simulink model "sddac"  (Simulink 5.0)
settings: Solver=ode45  StartTime=0.0  StopTime=10.0  RelTol=1e-3
values from neighbouring files (symbols this model uses):
  C = 680e-9    (= 6.8e-07)    [DPLL_init_2.m]    (also in pt8612_analog_pll_init.m = [1 0]; pt8612_analog_pll_init_2.m = [0 1 0]; pt8612_dpll_fpga_init.m; pt8612_dpll_fpga_init_2.m)
  Nbits = 16    [DPLL_init_2.m]    (also in pt8612_dpll_fpga_init.m; pt8612_dpll_fpga_init_2.m)
  R = 1/(wkneeloop*20)/C    (= 4060.30501089)    [DPLL_init_2.m]    (also in pt8612_dpll_fpga_init.m; pt8612_dpll_fpga_init_2.m = 3900)
  Tdac = 4/148.5e6    (= 2.6936026936e-08)    [DPLL_init_2.m]    (also in pt8612_dpll_fpga_init.m)
  Vvcxo0 = 1.25    [DPLL_init_2.m]    (also in pt8612_analog_pll_init.m; pt8612_analog_pll_init_2.m; pt8612_dpll_fpga_init.m; pt8612_dpll_fpga_init_2.m)
settings Model: LastModifiedBy=thh

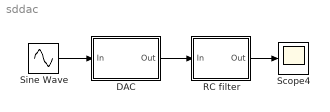
== system sddac ==
  DAC : Subsystem
  RC filter : Subsystem
  Scope4 : Scope
      settings: TimeRange=10  YMin=0.02  YMax=0.105
  Sine Wave : Sin  Amplitude=0.4  Bias=.5  Frequency=100  SampleTime=0
  wires:
  RC filter/1(Out) -> Scope4/1
  Sine Wave/1 -> DAC/1(In)
  DAC/1(Out) -> RC filter/1(In)

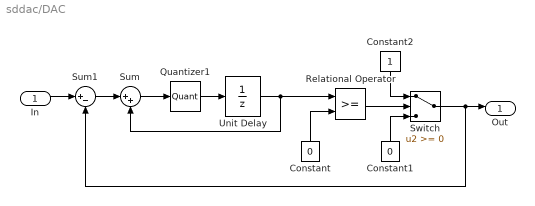
== system sddac/DAC ==
  In : Inport
  Constant : Constant  Orientation=up  Value=0
  Constant1 : Constant  Orientation=up  Value=0
  Constant2 : Constant  Orientation=down
  Quantizer1 : Quantizer  QuantizationInterval=2^-Nbits
  Relational Operator : RelationalOperator
  Sum : Sum  Inputs=|++  SaturateOnIntegerOverflow=on
  Sum1 : Sum  Inputs=|+-  SaturateOnIntegerOverflow=on
  Switch : Switch  SaturateOnIntegerOverflow=on
  Unit Delay : UnitDelay  SampleTime=Tdac
  Out : Outport
  wires:
  Sum/1 -> Quantizer1/1
  Unit Delay/1 -> Relational Operator/1, Sum/2
  Constant/1 -> Relational Operator/2
  Sum1/1 -> Sum/1
  Quantizer1/1 -> Unit Delay/1
  Relational Operator/1 -> Switch/2
  Constant1/1 -> Switch/3
  Constant2/1 -> Switch/1
  Switch/1 -> Sum1/2, Out/1
  In/1 -> Sum1/1

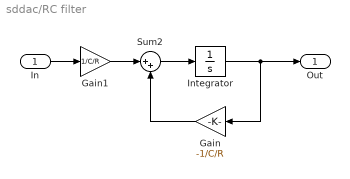
== system sddac/RC filter ==
  In : Inport
  Gain : Gain  Orientation=left  Gain=-1/C/R  SaturateOnIntegerOverflow=on
  Gain1 : Gain  Gain=1/C/R  SaturateOnIntegerOverflow=on
  Integrator : Integrator  InitialCondition=Vvcxo0
  Sum2 : Sum  Inputs=|++  SaturateOnIntegerOverflow=on
  Out : Outport
  wires:
  Gain1/1 -> Sum2/1
  Gain/1 -> Sum2/2
  Sum2/1 -> Integrator/1
  Integrator/1 -> Gain/1, Out/1
  In/1 -> Gain1/1
